simulink model "eval_condition"  (R2016b)
settings: Solver=ode1  StartTime=0.0  StopTime=100.0  FixedStep=0.001  RelTol=1e-3
values from neighbouring files (symbols this model uses):
  c1 = 0.004    [pid.m]    (also in pida.m; predictive_lqr.m)
  c12 = 0.017    [pid.m]    (also in pida.m; predictive_lqr.m)
  c2 = 0.05    [pid.m]    (also in pida.m; predictive_lqr.m)
  gr = 6*npd/npl    (= 4)    [pid.m]    (also in pida.m; predictive_lqr.m)
  Jdstr = Jd + Jp*grprime^(-2)    (= 0.00266925)    [pid.m]    (also in pida.m; predictive_lqr.m)
  Jl = Jdl + mwl*rwl^2 + Jwlo    (= 0.027125)    [pid.m]    (also in pida.m; predictive_lqr.m)
  k = 8.45    [pid.m]    (also in pida.m; predictive_lqr.m)
libraries: simulink x2
settings Model: Creator=davidshatwell  LastModifiedBy=davidshatwell

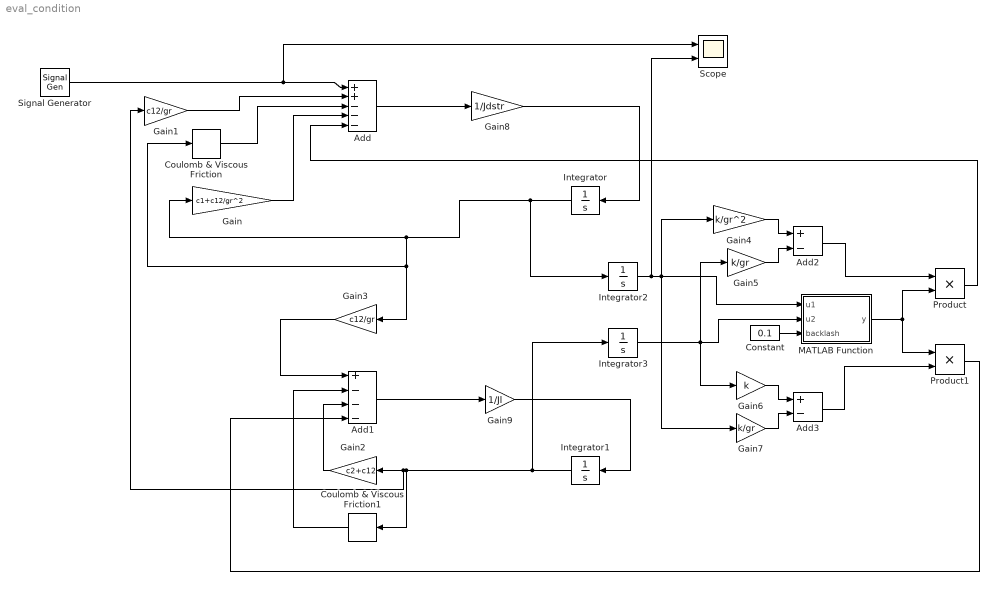
== system eval_condition ==
  Add : Sum  Inputs=++---
  Add1 : Sum  Inputs=+---
  Add2 : Sum  Inputs=+-
  Add3 : Sum  Inputs=+-
  Constant : Constant  Value=0.1
  Coulomb & Viscous Friction : simulink/Discontinuities/Coulomb & Viscous Friction  offset=0.1  gain=0
  Coulomb & Viscous Friction1 : simulink/Discontinuities/Coulomb & Viscous Friction  offset=0.1  gain=0
  Gain : Gain  Gain=c1+c12/gr^2
  Gain1 : Gain  Gain=c12/gr
  Gain2 : Gain  Gain=c2+c12
  Gain3 : Gain  Gain=c12/gr
  Gain4 : Gain  Gain=k/gr^2
  Gain5 : Gain  Gain=k/gr
  Gain6 : Gain  Gain=k
  Gain7 : Gain  Gain=k/gr
  Gain8 : Gain  Gain=1/Jdstr
  Gain9 : Gain  Gain=1/Jl
  Integrator{,1..3} (4 alike) : Integrator
  MATLAB Function : MATLAB Function  TreatAsAtomicUnit=on
  Product : Product
  Product1 : Product
  Scope : Scope  NumInputPorts=2
  Signal Generator : SignalGenerator  WaveForm=square  Frequency=1/50
  wires:
  Signal Generator/1 -> Scope/1, Add/1
  Integrator/1 -> Integrator2/1, Gain3/1, Coulomb & Viscous Friction/1, Gain/1
  Gain/1 -> Add/4
  Coulomb & Viscous Friction/1 -> Add/3
  Gain1/1 -> Add/2
  Integrator1/1 -> Gain2/1, Gain1/1, Coulomb & Viscous Friction1/1, Integrator3/1
  Gain2/1 -> Add1/3
  Coulomb & Viscous Friction1/1 -> Add1/2
  Gain3/1 -> Add1/1
  Integrator2/1 -> Scope/2, Gain7/1, Gain4/1, MATLAB Function/1(u1)
  Integrator3/1 -> Gain6/1, Gain5/1, MATLAB Function/2(u2)
  MATLAB Function/1(y) -> Product1/1, Product/2
  Gain4/1 -> Add2/1
  Gain5/1 -> Add2/2
  Add2/1 -> Product/1
  Gain6/1 -> Add3/1
  Gain7/1 -> Add3/2
  Add3/1 -> Product1/2
  Product/1 -> Add/5
  Product1/1 -> Add1/4
  Constant/1 -> MATLAB Function/3(backlash)
  Add/1 -> Gain8/1
  Gain8/1 -> Integrator/1
  Add1/1 -> Gain9/1
  Gain9/1 -> Integrator1/1

== matlab function eval_condition/MATLAB Function ==
  data: u1 input; y output; u2 input; backlash input
function y = fcn(u1, u2, backlash)

if (u2-u1 > 0) && (u2-u1 < backlash)
    y = false;
else
    y = true;
end

end
